simulink model "Stewart_simple"  (R2014a)
settings: Solver=ode3  SolverMode=SingleTasking  StartTime=0.0  StopTime=inf  RelTol=1e-3
StopFcn:
  | lecture
libraries: arduinolib x18, neural x6
settings Model: SimulationMode=external  CovModelRefEnable=off  CovSFcnEnable=on  ExtModeTrigDuration=2  Creator=costa  LastModifiedBy=rcostado
settings OptimizationCC: OptimizeModelRefInitCode=on  LifeSpan=1
settings DebuggingCC: UnderspecifiedInitializationDetection=Classic  SolverPrmCheckMsg=none
settings HardwareCC: ProdBitPerInt=16  ProdBitPerPointer=8  ProdIntDivRoundTo=Zero  ProdEndianess=LittleEndian  ProdWordSize=8  ProdHWDeviceType=Atmel->AVR
settings RTWCC: SystemTargetFile=realtime.tlc  GenerateMakefile=off  TemplateMakefile=realtime.tmf  Description=Run on Target Hardware  RTWVerbose=off  ProcessScript=realtime_make_rtw_hook
settings STFCustomTargetCC: TargetLibSuffix=.a  GenerateSampleERTMain=on  ConcurrentExecutionCompliant=off  GeneratePreprocessorConditionals=Use local settings  ERTCustomFileBanners=on  SupportNonInlinedSFcns=off  SupportVariableSizeSignals=on  MATLABClassNameForMDSCustomization=Simulink.SoftwareTarget.ERTCustomization  GRTInterface=off  SystemTargetFile=realtime.tlc
settings ERTTargetCC: CombineOutputUpdateFcns=off  SupportContinuousTime=on  SupportVariableSizeSignals=on  ExtModeTransport=3  ExtModeMexFile=ext_serial_win32_comm  ExtModeMexArgs=0 1 9600  ERTSrcFileBannerTemplate=realtime_code_template.cgt  ERTHdrFileBannerTemplate=realtime_code_template.cgt  ERTDataSrcFileTemplate=realtime_code_template.cgt  ERTDataHdrFileTemplate=realtime_code_template.cgt  ERTCustomFileTemplate=realtime_file_process.tlc

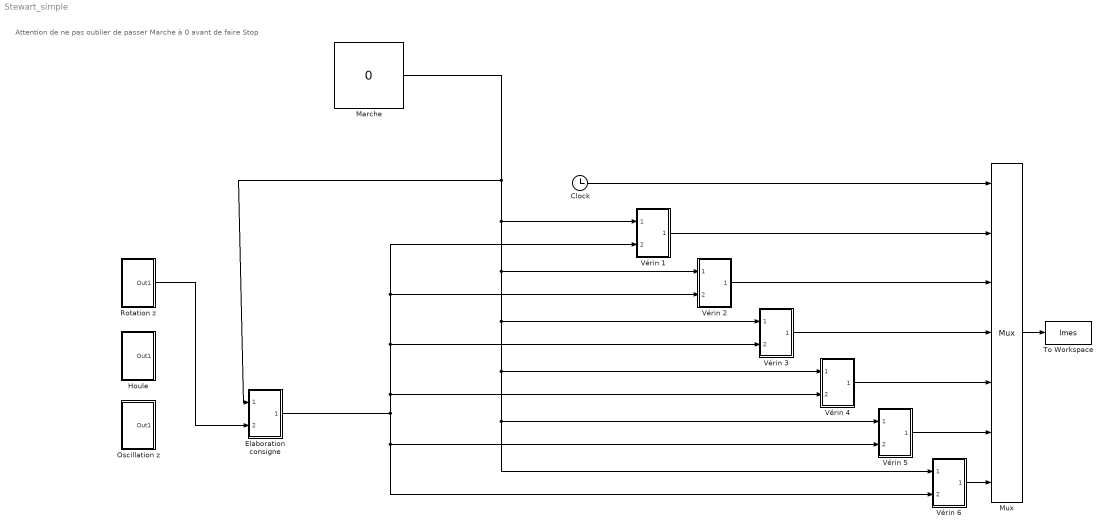
== system Stewart_simple ==
  note: Attention de ne pas oublier
      | de passer Marche à 0 avant de faire Stop
  Clock : Clock
  Elaboration consigne : Subsystem
  Houle : Subsystem
  Marche : Constant  Value=0
  Mux : Mux  Inputs=7
  Oscillation z : Subsystem
  Rotation z : Subsystem
  To Workspace : ToWorkspace  VariableName=lmes  SampleTime=-1
  Vérin 1 : Subsystem
  Vérin 2 : Subsystem
  Vérin 3 : Subsystem
  Vérin 4 : Subsystem
  Vérin 5 : Subsystem
  Vérin 6 : Subsystem
  wires:
  Marche/1 -> Vérin 6/1(In1), Vérin 5/1(In1), Vérin 4/1(In1), Vérin 3/1(In1), Vérin 2/1(In1), Vérin 1/1(In1), Elaboration consigne/1(In1)
  Mux/1 -> To Workspace/1
  Clock/1 -> Mux/1
  Vérin 1/1(Out1) -> Mux/2
  Vérin 2/1(Out1) -> Mux/3
  Vérin 3/1(Out1) -> Mux/4
  Vérin 4/1(Out1) -> Mux/5
  Vérin 5/1(Out1) -> Mux/6
  Vérin 6/1(Out1) -> Mux/7
  Elaboration consigne/1(Out1) -> Vérin 1/2(In2), Vérin 2/2(In2), Vérin 3/2(In2), Vérin 4/2(In2), Vérin 5/2(In2), Vérin 6/2(In2)
  Rotation z/1(Out1) -> Elaboration consigne/2(In2)

== system Stewart_simple/Elaboration consigne ==
  In1 : Inport
  In2 : Inport  Port=2
  Selecteur : Subsystem
  Switch6 : Switch  Criteria=u2 ~= 0
  To Workspace2 : ToWorkspace  VariableName=cons  SampleTime=-1
  Zero : Subsystem
  Out1 : Outport
  wires:
  In2/1 -> Switch6/1
  In1/1 -> Switch6/2
  Switch6/1 -> Selecteur/1(In2), To Workspace2/1
  Zero/1(Out1) -> Switch6/3
  Selecteur/1(Out1) -> Out1/1

== system Stewart_simple/Houle ==
  Mux1 : Mux  Inputs=6
  theta_x : Sin  Amplitude=pi/8  Frequency=40  SampleTime=0
  theta_y : Sin  Amplitude=pi/8  Frequency=40  Phase=pi/2  SampleTime=0
  theta_z : Constant  Value=0
  x : Constant  Value=0
  y : Constant  Value=0
  z : Constant  Value=0
  Out1 : Outport
  wires:
  theta_y/1 -> Mux1/2
  theta_z/1 -> Mux1/3
  y/1 -> Mux1/5
  theta_x/1 -> Mux1/1
  x/1 -> Mux1/4
  z/1 -> Mux1/6
  Mux1/1 -> Out1/1

== system Stewart_simple/Oscillation z ==
  Mux2 : Mux  Inputs=6
  theta_x : Constant  Value=0
  theta_y : Constant  Value=0
  theta_z : Constant  Value=0
  x : Constant  Value=0
  y : Constant  Value=0
  z : Sin  Amplitude=50  Frequency=60  SampleTime=0
  Out1 : Outport
  wires:
  z/1 -> Mux2/6
  x/1 -> Mux2/4
  theta_x/1 -> Mux2/1
  y/1 -> Mux2/5
  theta_z/1 -> Mux2/3
  theta_y/1 -> Mux2/2
  Mux2/1 -> Out1/1

== system Stewart_simple/Rotation z ==
  Mux1 : Mux  Inputs=6
  theta_x : Constant  Value=0
  theta_y : Constant  Value=0
  theta_z : Sin  Amplitude=pi/8  Frequency=100  SampleTime=0
  x : Constant  Value=0
  y : Constant  Value=0
  z : Constant  Value=0
  Out1 : Outport
  wires:
  theta_y/1 -> Mux1/2
  theta_z/1 -> Mux1/3
  y/1 -> Mux1/5
  theta_x/1 -> Mux1/1
  x/1 -> Mux1/4
  z/1 -> Mux1/6
  Mux1/1 -> Out1/1

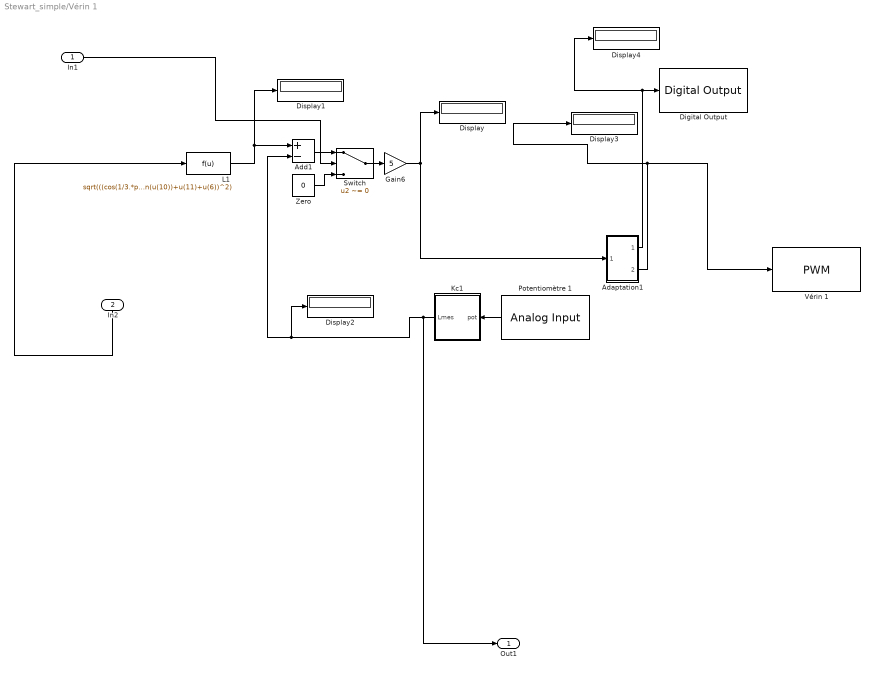
== system Stewart_simple/Vérin 1 ==
  In1 : Inport
  In2 : Inport  Port=2
  Adaptation1 : Subsystem
  Add1 : Sum  Inputs=+-
  Digital Output : arduinolib/Digital Output  pinNumber=11
  Display{,1..4} (5 alike) : Display
  Gain6 : Gain  Gain=5
  Kc1 : Subsystem
  L1 : Fcn  Expr=sqrt(((cos(1/3.*pi+u(3))*cos(u(2))-sin(1/3.*pi+u(3))*sin(u(1))*sin(u(2)))*u(7)*cos(u(10))+sin(1/3.*pi+u(3))*cos(u(1))*u(7)*sin(u(10))-u(8)*cos(u(9))+u(4))^2+ ((sin(1/3.*pi+u(3))*cos(u(2))+cos(1/3.*pi+u(3))*sin(u(1))*sin(u(2)))*u(7)*cos(u(10))-cos(1/3.*pi+u(3))*cos(u(1))*u(7)*sin(u(10))-u(8)*sin(u(9))+u(5))^2+ (-cos(u(1))*sin(u(2))*u(7)*cos(u(10))-sin(u(1))*u(7)*sin(u(10))+u(11)+u(6))^2)
  Potentiomètre 1 : arduinolib/Analog Input  pinNumber=2  sampleTime=0.001
  Switch : Switch  Criteria=u2 ~= 0
  Vérin 1 : arduinolib/PWM  pinNumber=10
  Zero : Constant  Value=0
  Out1 : Outport
  wires:
  In2/1 -> L1/1
  In1/1 -> Switch/2
  Potentiomètre 1/1 -> Kc1/1(pot)
  L1/1 -> Display1/1, Add1/1
  Gain6/1 -> Display/1, Adaptation1/1(ecart)
  Adaptation1/1(sens) -> Display4/1, Digital Output/1
  Adaptation1/2(pwm) -> Display3/1, Vérin 1/1
  Kc1/1(Lmes) -> Out1/1, Display2/1, Add1/2
  Switch/1 -> Gain6/1
  Add1/1 -> Switch/1
  Zero/1 -> Switch/3

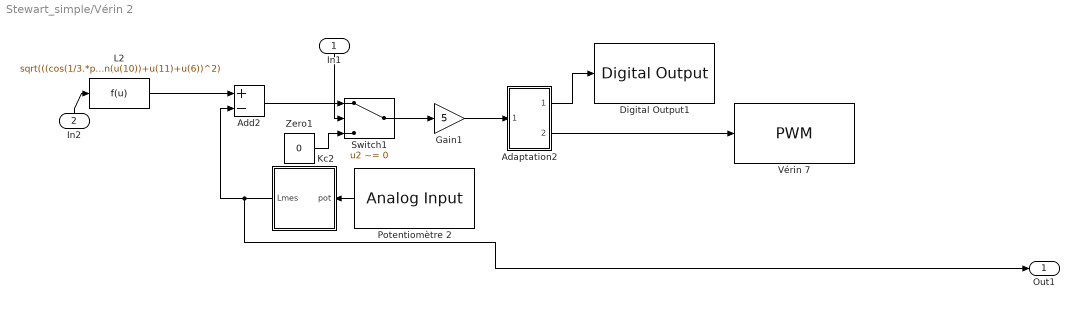
== system Stewart_simple/Vérin 2 ==
  In1 : Inport
  In2 : Inport  Port=2
  Adaptation2 : Subsystem
  Add2 : Sum  Inputs=+-
  Digital Output1 : arduinolib/Digital Output  pinNumber=5
  Gain1 : Gain  Gain=5
  Kc2 : Subsystem
  L2 : Fcn  Expr=sqrt(((cos(1/3.*pi+u(3))*cos(u(2))-sin(1/3.*pi+u(3))*sin(u(1))*sin(u(2)))*u(7)*cos(u(10))-sin(1/3.*pi+u(3))*cos(u(1))*u(7)*sin(u(10))+u(8)*cos(1/3.*pi+u(9))+u(4))^2+ ((sin(1/3.*pi+u(3))*cos(u(2))+cos(1/3.*pi+u(3))*sin(u(1))*sin(u(2)))*u(7)*cos(u(10))+cos(1/3.*pi+u(3))*cos(u(1))*u(7)*sin(u(10))-u(8)*sin(1/3.*pi+u(9))+u(5))^2+ (-cos(u(1))*sin(u(2))*u(7)*cos(u(10))+sin(u(1))*u(7)*sin(u(10))+u(11)+u(6))^2)
  Potentiomètre 2 : arduinolib/Analog Input  pinNumber=1  sampleTime=0.001
  Switch1 : Switch  Criteria=u2 ~= 0
  Vérin 7 : arduinolib/PWM  pinNumber=4
  Zero1 : Constant  Value=0
  Out1 : Outport
  wires:
  In1/1 -> Switch1/2
  In2/1 -> L2/1
  Gain1/1 -> Adaptation2/1(ecart)
  L2/1 -> Add2/1
  Adaptation2/1(sens) -> Digital Output1/1
  Adaptation2/2(pwm) -> Vérin 7/1
  Potentiomètre 2/1 -> Kc2/1(pot)
  Kc2/1(Lmes) -> Out1/1, Add2/2
  Add2/1 -> Switch1/1
  Switch1/1 -> Gain1/1
  Zero1/1 -> Switch1/3

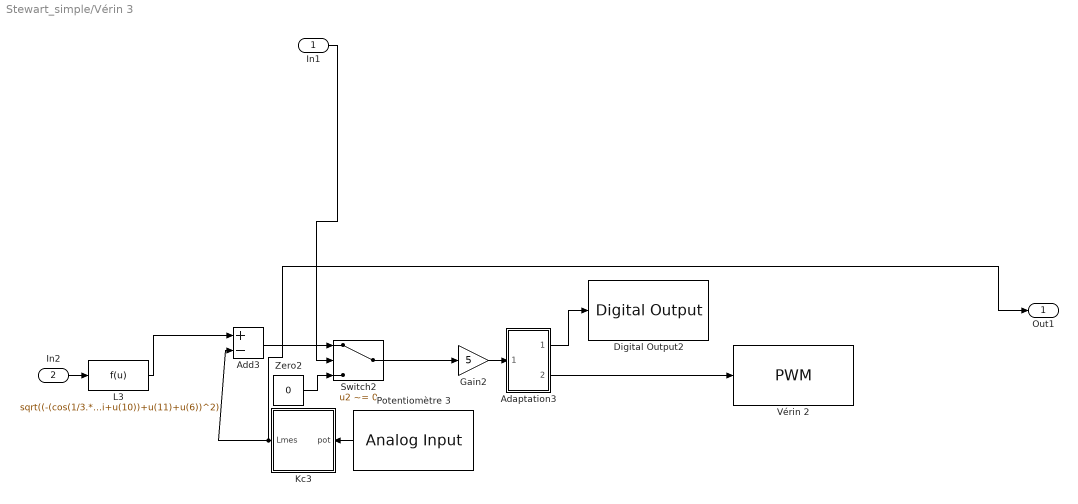
== system Stewart_simple/Vérin 3 ==
  In1 : Inport
  In2 : Inport  Port=2
  Adaptation3 : Subsystem
  Add3 : Sum  Inputs=+-
  Digital Output2 : arduinolib/Digital Output  pinNumber=3
  Gain2 : Gain  Gain=5
  Kc3 : Subsystem
  L3 : Fcn  Expr=sqrt((-(cos(1/3.*pi+u(3))*cos(u(2))-sin(1/3.*pi+u(3))*sin(u(1))*sin(u(2)))*u(7)*cos(1/3.*pi+u(10))-sin(1/3.*pi+u(3))*cos(u(1))*u(7)*sin(1/3.*pi+u(10))+u(8)*sin(1/6.*pi+u(9))+u(4))^2+(-(sin(1/3.*pi+u(3))*cos(u(2))+cos(1/3.*pi+u(3))*sin(u(1))*sin(u(2)))*u(7)*cos(1/3.*pi+u(10))+cos(1/3.*pi+u(3))*cos(u(1))*u(7)*sin(1/3.*pi+u(10))-u(8)*cos(1/6.*pi+u(9))+u(5))^2+(cos(u(1))*sin(u(2))*u(7)*cos(1/3.*pi+u(10))+sin(u(1))*u(7)*sin(1/3.*pi+u(10))+u(11)+u(6))^2)
  Potentiomètre 3 : arduinolib/Analog Input  pinNumber=0  sampleTime=0.001
  Switch2 : Switch  Criteria=u2 ~= 0
  Vérin 2 : arduinolib/PWM  pinNumber=2
  Zero2 : Constant  Value=0
  Out1 : Outport
  wires:
  In2/1 -> L3/1
  In1/1 -> Switch2/2
  L3/1 -> Add3/1
  Adaptation3/1(sens) -> Digital Output2/1
  Adaptation3/2(pwm) -> Vérin 2/1
  Gain2/1 -> Adaptation3/1(ecart)
  Potentiomètre 3/1 -> Kc3/1(pot)
  Kc3/1(Lmes) -> Out1/1, Add3/2
  Switch2/1 -> Gain2/1
  Zero2/1 -> Switch2/3
  Add3/1 -> Switch2/1

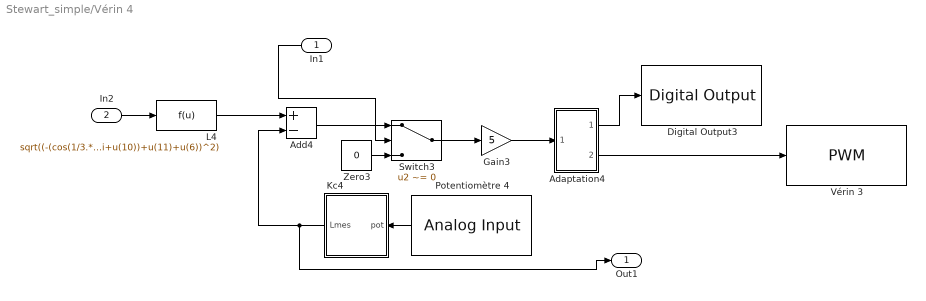
== system Stewart_simple/Vérin 4 ==
  In1 : Inport
  In2 : Inport  Port=2
  Adaptation4 : Subsystem
  Add4 : Sum  Inputs=+-
  Digital Output3 : arduinolib/Digital Output  pinNumber=9
  Gain3 : Gain  Gain=5
  Kc4 : Subsystem
  L4 : Fcn  Expr=sqrt((-(cos(1/3.*pi+u(3))*cos(u(2))-sin(1/3.*pi+u(3))*sin(u(1))*sin(u(2)))*u(7)*sin(1/6.*pi+u(10))-sin(1/3.*pi+u(3))*cos(u(1))*u(7)*cos(1/6.*pi+u(10))+u(8)*sin(1/6.*pi+u(9))+u(4))^2+(-(sin(1/3.*pi+u(3))*cos(u(2))+cos(1/3.*pi+u(3))*sin(u(1))*sin(u(2)))*u(7)*sin(1/6.*pi+u(10))+cos(1/3.*pi+u(3))*cos(u(1))*u(7)*cos(1/6.*pi+u(10))+u(8)*cos(1/6.*pi+u(9))+u(5))^2+(cos(u(1))*sin(u(2))*u(7)*sin(1/6.*pi+u(10))+sin(u(1))*u(7)*cos(1/6.*pi+u(10))+u(11)+u(6))^2)
  Potentiomètre 4 : arduinolib/Analog Input  pinNumber=5  sampleTime=0.001
  Switch3 : Switch  Criteria=u2 ~= 0
  Vérin 3 : arduinolib/PWM  pinNumber=8
  Zero3 : Constant  Value=0
  Out1 : Outport
  wires:
  In1/1 -> Switch3/2
  In2/1 -> L4/1
  L4/1 -> Add4/1
  Gain3/1 -> Adaptation4/1(ecart)
  Adaptation4/1(sens) -> Digital Output3/1
  Adaptation4/2(pwm) -> Vérin 3/1
  Kc4/1(Lmes) -> Out1/1, Add4/2
  Potentiomètre 4/1 -> Kc4/1(pot)
  Zero3/1 -> Switch3/3
  Switch3/1 -> Gain3/1
  Add4/1 -> Switch3/1

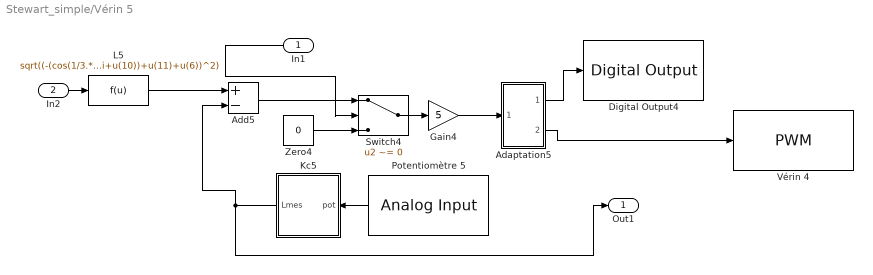
== system Stewart_simple/Vérin 5 ==
  In1 : Inport
  In2 : Inport  Port=2
  Adaptation5 : Subsystem
  Add5 : Sum  Inputs=+-
  Digital Output4 : arduinolib/Digital Output  pinNumber=7
  Gain4 : Gain  Gain=5
  Kc5 : Subsystem
  L5 : Fcn  Expr=sqrt((-(cos(1/3.*pi+u(3))*cos(u(2))-sin(1/3.*pi+u(3))*sin(u(1))*sin(u(2)))*u(7)*sin(1/6.*pi+u(10))+sin(1/3.*pi+u(3))*cos(u(1))*u(7)*cos(1/6.*pi+u(10))+u(8)*cos(1/3.*pi+u(9))+u(4))^2+(-(sin(1/3.*pi+u(3))*cos(u(2))+cos(1/3.*pi+u(3))*sin(u(1))*sin(u(2)))*u(7)*sin(1/6.*pi+u(10))-cos(1/3.*pi+u(3))*cos(u(1))*u(7)*cos(1/6.*pi+u(10))+u(8)*sin(1/3.*pi+u(9))+u(5))^2+(cos(u(1))*sin(u(2))*u(7)*sin(1/6.*pi+u(10))-sin(u(1))*u(7)*cos(1/6.*pi+u(10))+u(11)+u(6))^2)
  Potentiomètre 5 : arduinolib/Analog Input  pinNumber=4  sampleTime=0.001
  Switch4 : Switch  Criteria=u2 ~= 0
  Vérin 4 : arduinolib/PWM  pinNumber=6
  Zero4 : Constant  Value=0
  Out1 : Outport
  wires:
  In1/1 -> Switch4/2
  In2/1 -> L5/1
  L5/1 -> Add5/1
  Adaptation5/1(sens1) -> Digital Output4/1
  Adaptation5/2(pwm1) -> Vérin 4/1
  Potentiomètre 5/1 -> Kc5/1(pot)
  Kc5/1(Lmes) -> Out1/1, Add5/2
  Gain4/1 -> Adaptation5/1(ecart1)
  Switch4/1 -> Gain4/1
  Add5/1 -> Switch4/1
  Zero4/1 -> Switch4/3

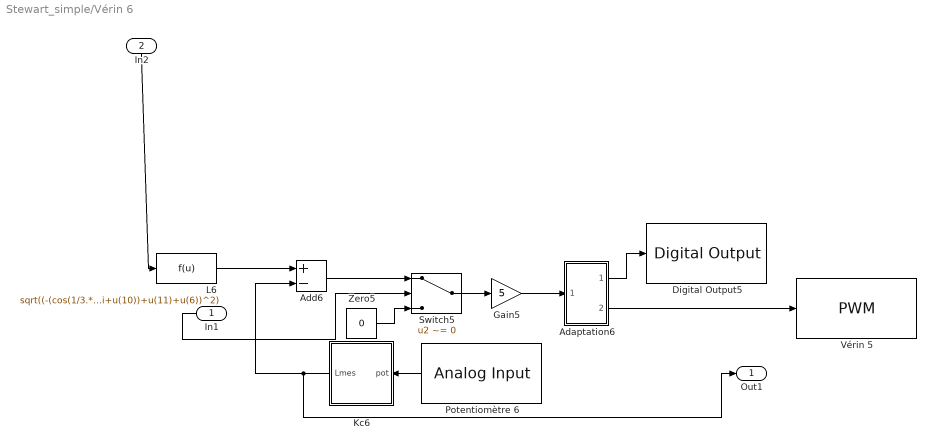
== system Stewart_simple/Vérin 6 ==
  In1 : Inport
  In2 : Inport  Port=2
  Adaptation6 : Subsystem
  Add6 : Sum  Inputs=+-
  Digital Output5 : arduinolib/Digital Output  pinNumber=13
  Gain5 : Gain  Gain=5
  Kc6 : Subsystem
  L6 : Fcn  Expr=sqrt((-(cos(1/3.*pi+u(3))*cos(u(2))-sin(1/3.*pi+u(3))*sin(u(1))*sin(u(2)))*u(7)*cos(1/3.*pi+u(10))+sin(1/3.*pi+u(3))*cos(u(1))*u(7)*sin(1/3.*pi+u(10))-u(8)*cos(u(9))+u(4))^2+(-(sin(1/3.*pi+u(3))*cos(u(2))+cos(1/3.*pi+u(3))*sin(u(1))*sin(u(2)))*u(7)*cos(1/3.*pi+u(10))-cos(1/3.*pi+u(3))*cos(u(1))*u(7)*sin(1/3.*pi+u(10))+u(8)*sin(u(9))+u(5))^2+(cos(u(1))*sin(u(2))*u(7)*cos(1/3.*pi+u(10))-sin(u(1))*u(7)*sin(1/3.*pi+u(10))+u(11)+u(6))^2)
  Potentiomètre 6 : arduinolib/Analog Input  pinNumber=3  sampleTime=0.001
  Switch5 : Switch  Criteria=u2 ~= 0
  Vérin 5 : arduinolib/PWM  pinNumber=12
  Zero5 : Constant  Value=0
  Out1 : Outport
  wires:
  In2/1 -> L6/1
  In1/1 -> Switch5/2
  L6/1 -> Add6/1
  Adaptation6/1(sens) -> Digital Output5/1
  Adaptation6/2(pwm) -> Vérin 5/1
  Potentiomètre 6/1 -> Kc6/1(pot)
  Kc6/1(Lmes) -> Out1/1, Add6/2
  Gain5/1 -> Adaptation6/1(ecart)
  Switch5/1 -> Gain5/1
  Zero5/1 -> Switch5/3
  Add6/1 -> Switch5/1

== system Stewart_simple/Elaboration consigne/Selecteur ==
  In2 : Inport
  Mux : Mux  Inputs=2
  Paramètres mécanisme : Subsystem
  Out1 : Outport
  wires:
  Paramètres mécanisme/1(Out1) -> Mux/2
  In2/1 -> Mux/1
  Mux/1 -> Out1/1

== system Stewart_simple/Elaboration consigne/Zero ==
  Mux1 : Mux  Inputs=6
  theta_x1 : Constant  Value=0
  theta_y1 : Constant  Value=0
  theta_z1 : Constant  Value=0
  x1 : Constant  Value=0
  y1 : Constant  Value=0
  z1 : Constant  Value=0
  Out1 : Outport
  wires:
  Mux1/1 -> Out1/1
  theta_y1/1 -> Mux1/2
  theta_z1/1 -> Mux1/3
  y1/1 -> Mux1/5
  theta_x1/1 -> Mux1/1
  x1/1 -> Mux1/4
  z1/1 -> Mux1/6

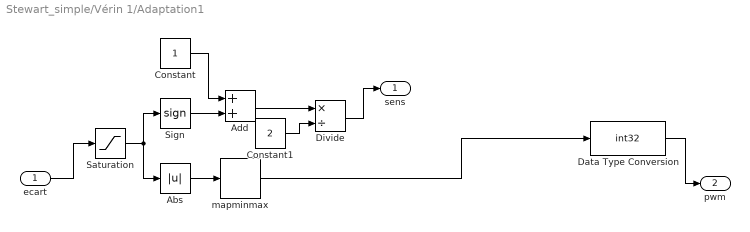
== system Stewart_simple/Vérin 1/Adaptation1 ==
  ecart : Inport
  Abs : Abs
  Add : Sum
  Constant : Constant
  Constant1 : Constant  Value=2
  Data Type Conversion : DataTypeConversion  OutDataTypeStr=int32
  Divide : Product  Inputs=*/
  Saturation : Saturate  UpperLimit=200  LowerLimit=-200
  Sign : Signum
  mapminmax : neural/Processing Functions/mapminmax  xmin=0  xmax=200  ymin=1  ymax=255
  sens : Outport
  pwm : Outport  Port=2
  wires:
  ecart/1 -> Saturation/1
  Abs/1 -> mapminmax/1
  Saturation/1 -> Sign/1, Abs/1
  Sign/1 -> Add/2
  Constant/1 -> Add/1
  Add/1 -> Divide/1
  Constant1/1 -> Divide/2
  Divide/1 -> sens/1
  Data Type Conversion/1 -> pwm/1
  mapminmax/1 -> Data Type Conversion/1

== system Stewart_simple/Vérin 1/Kc1 ==
  pot : Inport
  Add : Sum  Inputs=-+
  Add1 : Sum
  Divide : Product  Inputs=**
  Gain1 : Gain  Gain=1/1024
  Lmax : Constant  Value=500
  Lmin : Constant  Value=350
  Lmes : Outport
  wires:
  Lmin/1 -> Add1/1, Add/1
  Lmax/1 -> Add/2
  Gain1/1 -> Divide/2
  Divide/1 -> Add1/2
  Add1/1 -> Lmes/1
  pot/1 -> Gain1/1
  Add/1 -> Divide/1

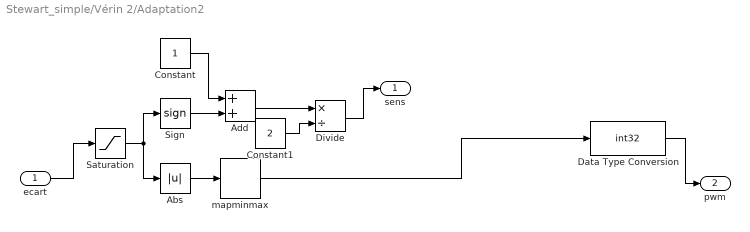
== system Stewart_simple/Vérin 2/Adaptation2 ==
  ecart : Inport
  Abs : Abs
  Add : Sum
  Constant : Constant
  Constant1 : Constant  Value=2
  Data Type Conversion : DataTypeConversion  OutDataTypeStr=int32
  Divide : Product  Inputs=*/
  Saturation : Saturate  UpperLimit=200  LowerLimit=-200
  Sign : Signum
  mapminmax : neural/Processing Functions/mapminmax  xmin=0  xmax=200  ymin=1  ymax=255
  sens : Outport
  pwm : Outport  Port=2
  wires:
  ecart/1 -> Saturation/1
  Abs/1 -> mapminmax/1
  Saturation/1 -> Sign/1, Abs/1
  Sign/1 -> Add/2
  Constant/1 -> Add/1
  Add/1 -> Divide/1
  Constant1/1 -> Divide/2
  Divide/1 -> sens/1
  Data Type Conversion/1 -> pwm/1
  mapminmax/1 -> Data Type Conversion/1

== system Stewart_simple/Vérin 2/Kc2 ==
  pot : Inport
  Add : Sum  Inputs=-+
  Add1 : Sum
  Divide : Product  Inputs=**
  Gain1 : Gain  Gain=1/1024
  Lmax : Constant  Value=500
  Lmin : Constant  Value=350
  Lmes : Outport
  wires:
  Lmin/1 -> Add1/1, Add/1
  Lmax/1 -> Add/2
  Gain1/1 -> Divide/2
  Divide/1 -> Add1/2
  Add1/1 -> Lmes/1
  pot/1 -> Gain1/1
  Add/1 -> Divide/1

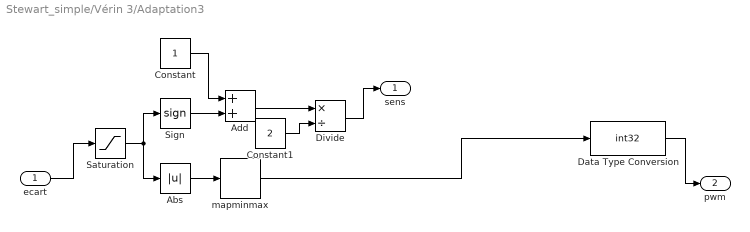
== system Stewart_simple/Vérin 3/Adaptation3 ==
  ecart : Inport
  Abs : Abs
  Add : Sum
  Constant : Constant
  Constant1 : Constant  Value=2
  Data Type Conversion : DataTypeConversion  OutDataTypeStr=int32
  Divide : Product  Inputs=*/
  Saturation : Saturate  UpperLimit=200  LowerLimit=-200
  Sign : Signum
  mapminmax : neural/Processing Functions/mapminmax  xmin=0  xmax=200  ymin=1  ymax=255
  sens : Outport
  pwm : Outport  Port=2
  wires:
  ecart/1 -> Saturation/1
  Abs/1 -> mapminmax/1
  Saturation/1 -> Sign/1, Abs/1
  Sign/1 -> Add/2
  Constant/1 -> Add/1
  Add/1 -> Divide/1
  Constant1/1 -> Divide/2
  Divide/1 -> sens/1
  Data Type Conversion/1 -> pwm/1
  mapminmax/1 -> Data Type Conversion/1

== system Stewart_simple/Vérin 3/Kc3 ==
  pot : Inport
  Add : Sum  Inputs=-+
  Add1 : Sum
  Divide : Product  Inputs=**
  Gain1 : Gain  Gain=1/1024
  Lmax : Constant  Value=500
  Lmin : Constant  Value=350
  Lmes : Outport
  wires:
  Lmin/1 -> Add1/1, Add/1
  Lmax/1 -> Add/2
  Gain1/1 -> Divide/2
  Divide/1 -> Add1/2
  Add1/1 -> Lmes/1
  pot/1 -> Gain1/1
  Add/1 -> Divide/1

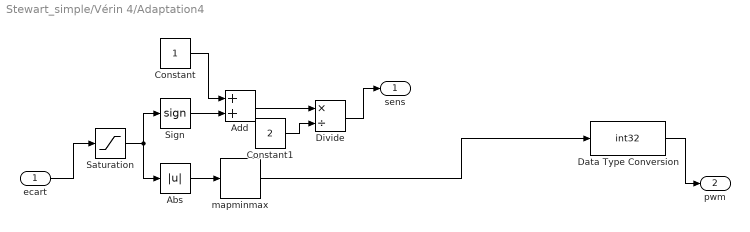
== system Stewart_simple/Vérin 4/Adaptation4 ==
  ecart : Inport
  Abs : Abs
  Add : Sum
  Constant : Constant
  Constant1 : Constant  Value=2
  Data Type Conversion : DataTypeConversion  OutDataTypeStr=int32
  Divide : Product  Inputs=*/
  Saturation : Saturate  UpperLimit=200  LowerLimit=-200
  Sign : Signum
  mapminmax : neural/Processing Functions/mapminmax  xmin=0  xmax=200  ymin=1  ymax=255
  sens : Outport
  pwm : Outport  Port=2
  wires:
  ecart/1 -> Saturation/1
  Abs/1 -> mapminmax/1
  Saturation/1 -> Sign/1, Abs/1
  Sign/1 -> Add/2
  Constant/1 -> Add/1
  Add/1 -> Divide/1
  Constant1/1 -> Divide/2
  Divide/1 -> sens/1
  Data Type Conversion/1 -> pwm/1
  mapminmax/1 -> Data Type Conversion/1

== system Stewart_simple/Vérin 4/Kc4 ==
  pot : Inport
  Add : Sum  Inputs=-+
  Add1 : Sum
  Divide : Product  Inputs=**
  Gain1 : Gain  Gain=1/1024
  Lmax : Constant  Value=500
  Lmin : Constant  Value=350
  Lmes : Outport
  wires:
  Lmin/1 -> Add1/1, Add/1
  Lmax/1 -> Add/2
  Gain1/1 -> Divide/2
  Divide/1 -> Add1/2
  Add1/1 -> Lmes/1
  pot/1 -> Gain1/1
  Add/1 -> Divide/1

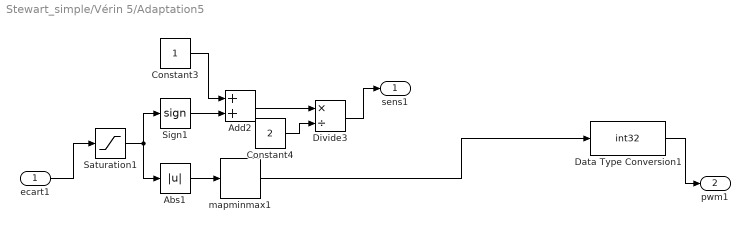
== system Stewart_simple/Vérin 5/Adaptation5 ==
  ecart1 : Inport
  Abs1 : Abs
  Add2 : Sum
  Constant3 : Constant
  Constant4 : Constant  Value=2
  Data Type Conversion1 : DataTypeConversion  OutDataTypeStr=int32
  Divide3 : Product  Inputs=*/
  Saturation1 : Saturate  UpperLimit=200  LowerLimit=-200
  Sign1 : Signum
  mapminmax1 : neural/Processing Functions/mapminmax  xmin=0  xmax=200  ymin=1  ymax=255
  sens1 : Outport
  pwm1 : Outport  Port=2
  wires:
  ecart1/1 -> Saturation1/1
  Abs1/1 -> mapminmax1/1
  Saturation1/1 -> Sign1/1, Abs1/1
  Sign1/1 -> Add2/2
  Constant3/1 -> Add2/1
  Add2/1 -> Divide3/1
  Constant4/1 -> Divide3/2
  Divide3/1 -> sens1/1
  Data Type Conversion1/1 -> pwm1/1
  mapminmax1/1 -> Data Type Conversion1/1

== system Stewart_simple/Vérin 5/Kc5 ==
  pot : Inport
  Add : Sum  Inputs=-+
  Add1 : Sum
  Divide : Product  Inputs=**
  Gain1 : Gain  Gain=1/1024
  Lmax : Constant  Value=500
  Lmin : Constant  Value=350
  Lmes : Outport
  wires:
  Lmin/1 -> Add1/1, Add/1
  Lmax/1 -> Add/2
  Gain1/1 -> Divide/2
  Divide/1 -> Add1/2
  Add1/1 -> Lmes/1
  pot/1 -> Gain1/1
  Add/1 -> Divide/1

== system Stewart_simple/Vérin 6/Adaptation6 ==
  ecart : Inport
  Abs : Abs
  Add : Sum
  Constant : Constant
  Constant1 : Constant  Value=2
  Data Type Conversion : DataTypeConversion  OutDataTypeStr=int32
  Divide : Product  Inputs=*/
  Saturation : Saturate  UpperLimit=200  LowerLimit=-200
  Sign : Signum
  mapminmax : neural/Processing Functions/mapminmax  xmin=0  xmax=200  ymin=1  ymax=255
  sens : Outport
  pwm : Outport  Port=2
  wires:
  ecart/1 -> Saturation/1
  Abs/1 -> mapminmax/1
  Saturation/1 -> Sign/1, Abs/1
  Sign/1 -> Add/2
  Constant/1 -> Add/1
  Add/1 -> Divide/1
  Constant1/1 -> Divide/2
  Divide/1 -> sens/1
  Data Type Conversion/1 -> pwm/1
  mapminmax/1 -> Data Type Conversion/1

== system Stewart_simple/Vérin 6/Kc6 ==
  pot : Inport
  Add : Sum  Inputs=-+
  Add1 : Sum
  Divide : Product  Inputs=**
  Gain1 : Gain  Gain=1/1024
  Lmax : Constant  Value=500
  Lmin : Constant  Value=350
  Lmes : Outport
  wires:
  Lmin/1 -> Add1/1, Add/1
  Lmax/1 -> Add/2
  Gain1/1 -> Divide/2
  Divide/1 -> Add1/2
  Add1/1 -> Lmes/1
  pot/1 -> Gain1/1
  Add/1 -> Divide/1

== system Stewart_simple/Elaboration consigne/Selecteur/Paramètres mécanisme ==
  Mux1 : Mux  Inputs=5
  alpha : Constant  Value=0.007
  beta : Constant  Value=0.009
  h : Constant  Value=380
  rf : Constant  Value=270
  rm : Constant  Value=200
  Out1 : Outport
  wires:
  Mux1/1 -> Out1/1
  rm/1 -> Mux1/1
  rf/1 -> Mux1/2
  alpha/1 -> Mux1/3
  beta/1 -> Mux1/4
  h/1 -> Mux1/5
